simulink model "sfcndemo_dtype_param"  (Simulink 7.6)
settings: Solver=FixedStepDiscrete  StartTime=0.0  StopTime=10.0  RelTol=1e-3
Description:
  | Data-Typed Parameter Handling in C-MEX S-functions
settings Model: Creator=The MathWorks Inc.  ExtModeAutoUpdateStatusClock=off
settings OptimizationCC: BlockReduction=off  BooleanDataType=off  InitFltsAndDblsToZero=on
settings DebuggingCC: SaveWithParameterizedLinksMsg=none  SignalResolutionControl=TryResolveAllWithWarning  SolverPrmCheckMsg=none  MultiTaskDSMMsg=warning  MultiTaskCondExecSysMsg=none
settings HardwareCC: TargetUnknown=on
settings RTWCC: IncludeERTFirstTime=on
settings CodeAppCC: CustomSymbolStrFcn=$F$N$M
settings GRTTargetCC: TargetFcnLib=ansi_tfl_tmw.mat

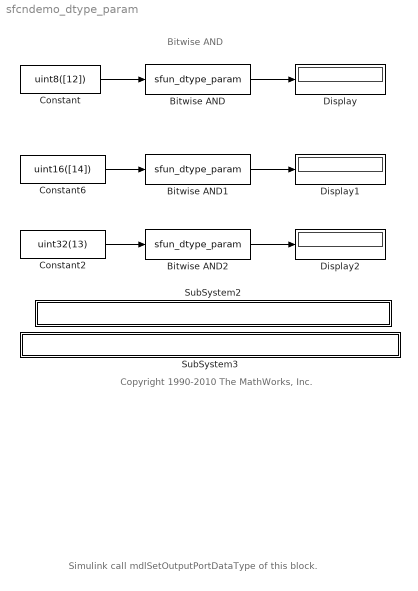
== system sfcndemo_dtype_param ==
  note: Simulink call mdlSetOutputPortDataType of this block.
  note: Bitwise AND
  note: Copyright 1990-2010 The MathWorks, Inc.
  Bitwise AND : S-Function  FunctionName=sfun_dtype_param  Parameters=uint8(11)  EnableBusSupport=off
      settings: AttributesFormatString=%<Parameters>
  Bitwise AND1 : S-Function  FunctionName=sfun_dtype_param  Parameters=uint16(7)  EnableBusSupport=off
      settings: AttributesFormatString=%<Parameters>
  Bitwise AND2 : S-Function  FunctionName=sfun_dtype_param  Parameters=uint32(6)  EnableBusSupport=off
      settings: AttributesFormatString=%<Parameters>
  Constant : Constant  Value=uint8([12])
  Constant2 : Constant  Value=uint32(13)
  Constant6 : Constant  Value=uint16([14])
  Display : Display
  Display1 : Display
  Display2 : Display
  SubSystem2 : Subsystem  mask{filename=sfun_dtype_param.c}
      mask init:
      | x=sfundemo_maskdisp;
      settings: AttributesFormatString=\n  OpenFcn=sfundemo_openfcn
      mask Display: disp(x);
  SubSystem3 : Subsystem  mask{filename=sfun_dtype_param.tlc}
      mask init:
      | x=sfundemo_maskdisp;
      settings: AttributesFormatString=\n  OpenFcn=sfundemo_openfcn
      mask Display: disp(x);
  wires:
  Constant/1 -> Bitwise AND/1
  Bitwise AND/1 -> Display/1
  Constant6/1 -> Bitwise AND1/1
  Bitwise AND1/1 -> Display1/1
  Constant2/1 -> Bitwise AND2/1
  Bitwise AND2/1 -> Display2/1

== system sfcndemo_dtype_param/SubSystem2 ==

== system sfcndemo_dtype_param/SubSystem3 ==
